simulink model "UDPConnection2"  (R2022b)
settings: configuration reference "WheelSimConfiguration" (kept outside this file)
libraries: slrealtimeutilitieslib x2, slrealtimeiplib x2
settings Model: Creator=ateay  LastModifiedBy=MOSA
settings ConfigSetRef: SourceName=WheelSimConfiguration  SourceLocation=Base Workspace

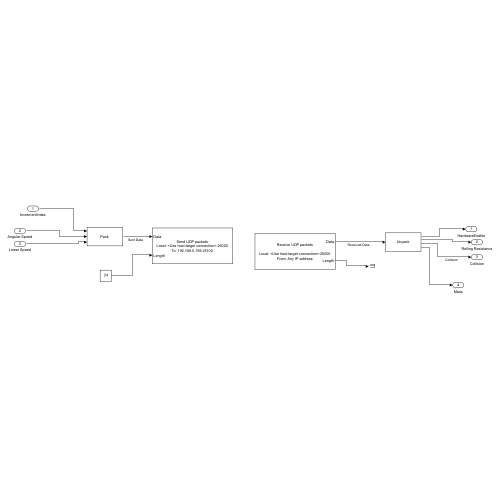
[thumbnail: Simulink's stored preview of the top-level diagram]
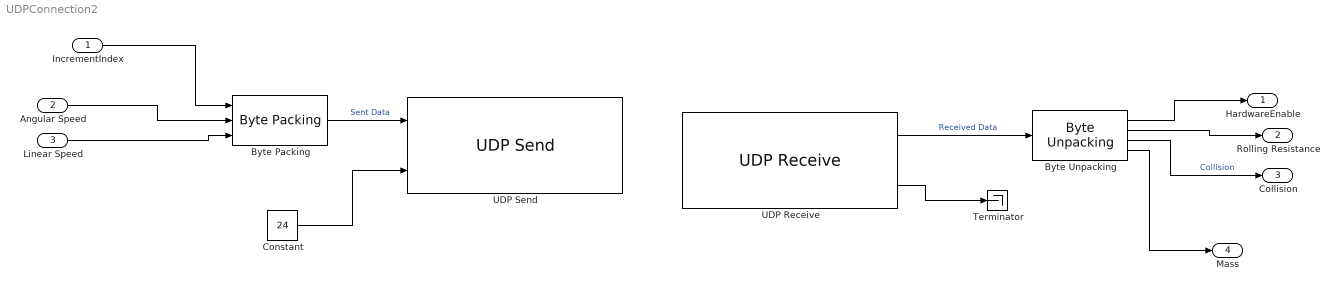
== system UDPConnection2 ==
  IncrementIndex : Inport
  Angular Speed : Inport  Port=2
  Linear Speed : Inport  Port=3
  Byte Packing : slrealtimeutilitieslib/Byte Packing  MaskPackedDataType=uint8  MaskUnpackedDataTypes={['double'],['double'],['double']}  MaskAlignment=1
  Byte Unpacking : slrealtimeutilitieslib/Byte Unpacking  MaskUnpackedDataTypes={['double'],['double'],'boolean',['double']}  MaskUnpackedDataSizes={[1] [1] [1] [1]}  MaskAlignment=4
  Constant : Constant  Value=24
  Terminator : Terminator
  UDP Receive : slrealtimeiplib/UDP Receive  useHostTargetConn=on  ipAddress=192.168.0.200  localPort=25000  rcvWidth=28  rcvFmAny=on  fmAddress=192.168.0.2  sampleTime=simulator.TimeStep  enableMessage=off  maxPackets=1
  UDP Send : slrealtimeiplib/UDP Send  useHostTargetConn=on  toAddress=192.168.0.159  toPort=25100  sampleTime=simulator.TimeStep  enableMessage=off  ipAddress=192.168.0.200  localPort=25000
  HardwareEnable : Outport
  Rolling Resistance : Outport  Port=2
  Collision : Outport  Port=3
  Mass : Outport  Port=4
  wires:
  Byte Packing/1 -> UDP Send/1  "Sent Data"
  Angular Speed/1 -> Byte Packing/2
  Linear Speed/1 -> Byte Packing/3
  UDP Receive/1 -> Byte Unpacking/1  "Received Data"
  Constant/1 -> UDP Send/2
  UDP Receive/2 -> Terminator/1
  Byte Unpacking/2 -> Rolling Resistance/1
  Byte Unpacking/3 -> Collision/1  "Collision"
  IncrementIndex/1 -> Byte Packing/1
  Byte Unpacking/1 -> HardwareEnable/1
  Byte Unpacking/4 -> Mass/1
